simulink model "Valve_Test"  (R2024b)
settings: Solver=VariableStepAuto  StartTime=0.0  StopTime=10.0  RelTol=1e-3
values from neighbouring files (symbols this model uses):
  c1 = 1.27e-7    (= 1.27e-07)    [Caculation.m]
  c2 = 6.37e-8    (= 6.37e-08)    [Caculation.m]
  kv = 0.15    [Caculation.m]
  rio_H2 = 0.089    [Caculation.m]
settings Model: Creator=10537  LastModifiedBy=10537

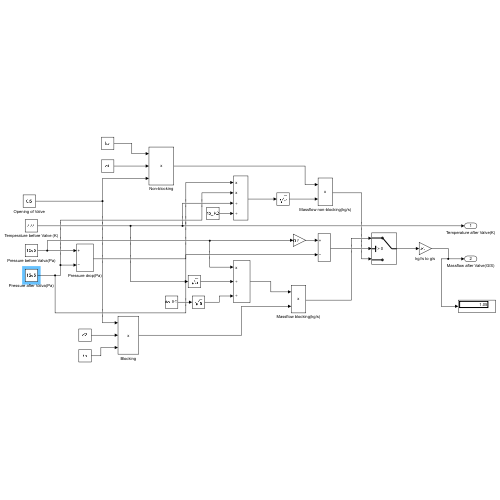
[thumbnail: Simulink's stored preview of the top-level diagram]
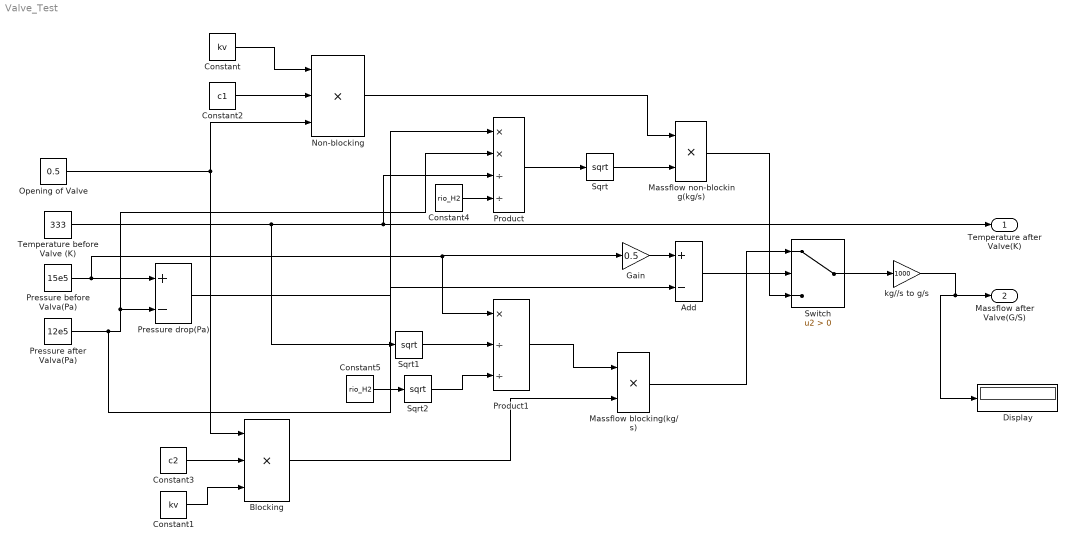
== system Valve_Test ==
  Add : Sum  Inputs=+-
  Blocking : Product  Inputs=3
  Constant : Constant  Value=kv
  Constant1 : Constant  Value=kv
  Constant2 : Constant  Value=c1
  Constant3 : Constant  Value=c2
  Constant4 : Constant  Value=rio_H2
  Constant5 : Constant  Value=rio_H2
  Display : Display
  Gain : Gain  Gain=0.5
  Massflow blocking(kg/s) : Product
  Massflow non-blocking(kg/s) : Product
  Non-blocking : Product  Inputs=3
  Opening of Valve : Constant  Value=0.5
  Pressure after Valva(Pa) : Constant  Value=12e5
  Pressure before Valva(Pa) : Constant  Value=15e5
  Pressure drop(Pa) : Sum  Inputs=+-
  Product : Product  Inputs=**//
  Product1 : Product  Inputs=*//
  Sqrt : Sqrt
  Sqrt1 : Sqrt
  Sqrt2 : Sqrt
  Switch : Switch  Criteria=u2 > Threshold  SaturateOnIntegerOverflow=off  InputSameDT=off
  Temperature before Valve (K) : Constant  Value=333
  kg//s to g/s : Gain  Gain=1000
  Temperature after Valve(K) : Outport
  Massflow after Valve(G/S) : Outport  Port=2
  wires:
  Temperature before Valve (K)/1 -> Sqrt1/1, Product/3, Temperature after Valve(K)/1
  Opening of Valve/1 -> Blocking/1, Non-blocking/3
  Constant/1 -> Non-blocking/1
  Constant2/1 -> Non-blocking/2
  Constant3/1 -> Blocking/2
  Constant1/1 -> Blocking/3
  Pressure before Valva(Pa)/1 -> Product1/1, Gain/1, Pressure drop(Pa)/1
  Pressure after Valva(Pa)/1 -> Add/2, Product/2, Pressure drop(Pa)/2
  Pressure drop(Pa)/1 -> Product/1
  Constant4/1 -> Product/4
  Product/1 -> Sqrt/1
  Sqrt/1 -> Massflow non-blocking(kg/s)/2
  Non-blocking/1 -> Massflow non-blocking(kg/s)/1
  Constant5/1 -> Sqrt2/1
  Sqrt2/1 -> Product1/3
  Sqrt1/1 -> Product1/2
  Product1/1 -> Massflow blocking(kg/s)/1
  Blocking/1 -> Massflow blocking(kg/s)/2
  Gain/1 -> Add/1
  Add/1 -> Switch/2
  Massflow blocking(kg/s)/1 -> Switch/1
  Massflow non-blocking(kg/s)/1 -> Switch/3
  Switch/1 -> kg//s to g/s/1
  kg//s to g/s/1 -> Massflow after Valve(G/S)/1, Display/1
